simulink model "aerodynamic_hopper"  (R2022b)
settings: Solver=VariableStepAuto  StartTime=0.0  StopTime=1  RelTol=1e-3
libraries: aerolibadyn x1, sharedtransform x1, aerolibasang x1, aerolibatmos2 x1
settings Model: Creator=ks  LastModifiedBy=User
settings OptimizationCC: ReuseModelBlockBuffer=on
settings RTWCC: GPUComputeCapability=5.0

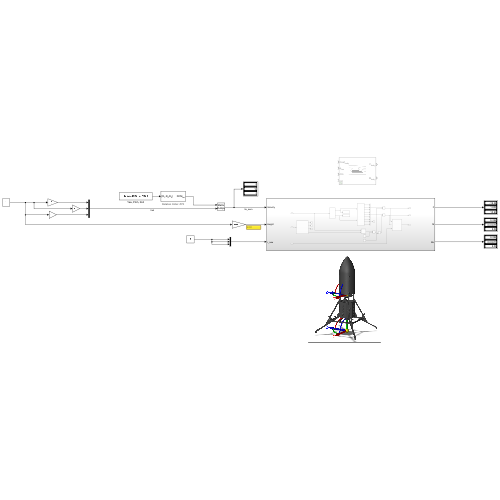
[thumbnail: Simulink's stored preview of the top-level diagram]
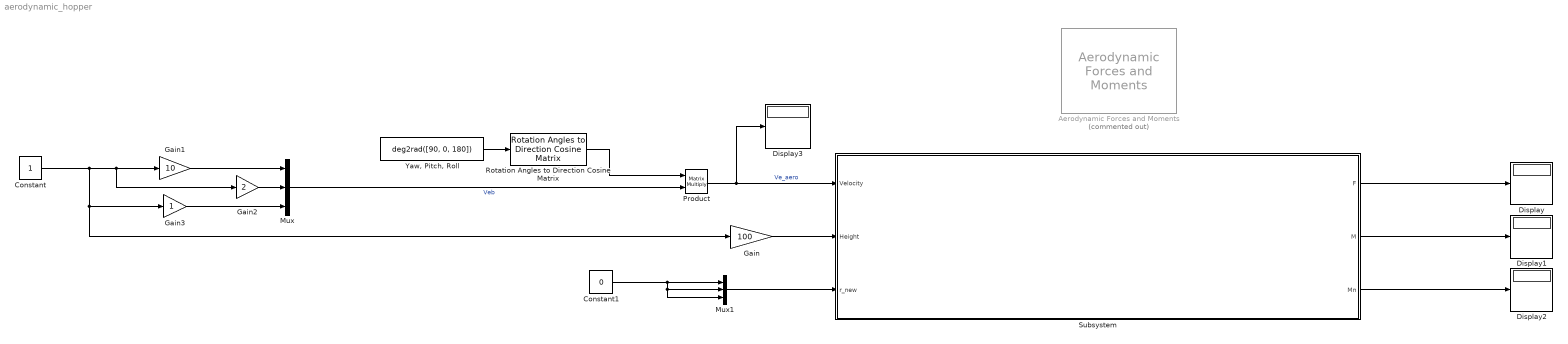
== system aerodynamic_hopper ==
  "Aerodynamic Forces and Moments " : aerolibadyn/Aerodynamic Forces and Moments   Commented=on  inputAxes=Body  outputForceAxes=Body  outputMomentAxes=Body  S=1  b=1  cbar=1
  Constant : Constant
  Constant1 : Constant  Value=0
  Display{,1..3} (4 alike) : Display
  Gain : Gain  Gain=100
  Gain1 : Gain  Gain=10
  Gain2 : Gain  Gain=2
  Gain3 : Gain
  Mux : Mux  Inputs=3
  Mux1 : Mux  Inputs=3
  Product : Product  Multiplication=Matrix(*)
  Rotation Angles to Direction Cosine Matrix : sharedtransform/Rotation Angles to Direction Cosine Matrix  rotationOrder=ZYX  aMode=aMode
  Subsystem : Subsystem
  "Yaw, Pitch, Roll" : Constant  Value=deg2rad([90, 0, 180])
  wires:
  Constant/1 -> Gain1/1, Gain2/1, Gain3/1, Gain/1
  Mux1/1 -> Subsystem/3(r_new)
  Subsystem/1(F) -> Display/1
  Subsystem/2(M) -> Display1/1
  Subsystem/3(Mn) -> Display2/1
  Mux/1 -> Product/2  "Veb"
  Gain/1 -> Subsystem/2(Height)
  Gain1/1 -> Mux/1
  Gain2/1 -> Mux/2
  Constant1/1 -> Mux1/3, Mux1/2, Mux1/1
  "Yaw, Pitch, Roll"/1 -> Rotation Angles to Direction Cosine Matrix/1
  Product/1 -> Display3/1, Subsystem/1(Velocity)  "Ve_aero"
  Rotation Angles to Direction Cosine Matrix/1 -> Product/1
  Gain3/1 -> Mux/3

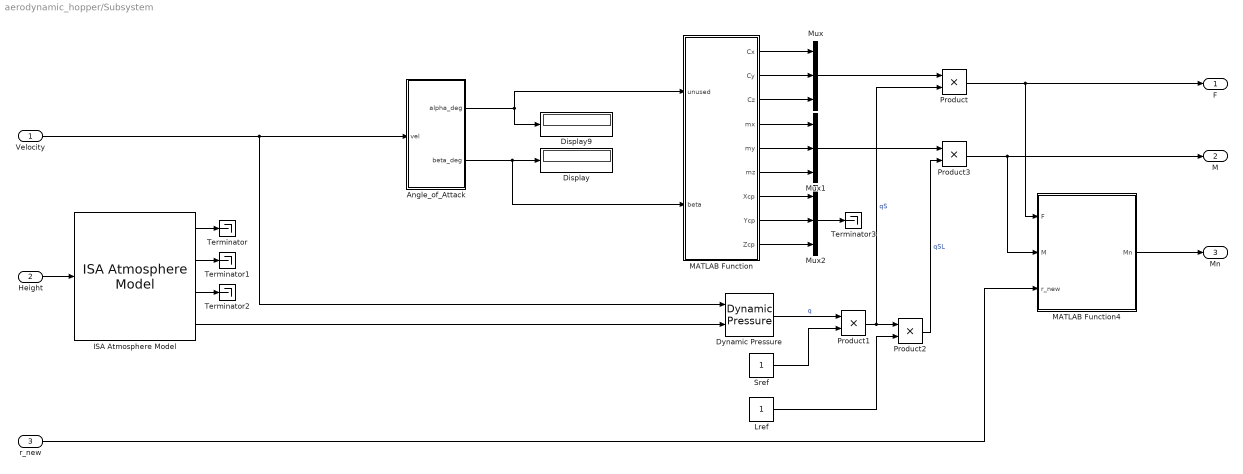
== system aerodynamic_hopper/Subsystem ==
  Velocity : Inport
  Height : Inport  Port=2
  r_new : Inport  Port=3
  Angle_of_Attack : MATLAB Function  TreatAsAtomicUnit=on
  Display : Display
  Display9 : Display
  Dynamic Pressure : aerolibasang/Dynamic Pressure
  ISA Atmosphere Model : aerolibatmos2/ISA Atmosphere Model  custom=off  g=9.80665  gamma=1.4  R=287.0531  L=0.0065  h_trop=11000  h_strat=20000  rho0=1.225  P0=101325  T0=288.15  h0=0
  Lref : Constant
  MATLAB Function : MATLAB Function  TreatAsAtomicUnit=on
  MATLAB Function4 : MATLAB Function  TreatAsAtomicUnit=on
  Mux : Mux  Inputs=3
  Mux1 : Mux  Inputs=3
  Mux2 : Mux  Inputs=3
  Product{,1..3} (4 alike) : Product
  Sref : Constant
  Terminator{,1..3} (4 alike) : Terminator
  F : Outport
  M : Outport  Port=2
  Mn : Outport  Port=3
  wires:
  Mux2/1 -> Terminator3/1
  ISA Atmosphere Model/4 -> Dynamic Pressure/2
  Angle_of_Attack/1(alpha_deg) -> Display9/1, MATLAB Function/1(unused)
  Product/1 -> F/1, MATLAB Function4/1(F)
  MATLAB Function/7(Xcp) -> Mux2/1
  Velocity/1 -> Dynamic Pressure/1, Angle_of_Attack/1(vel)
  Sref/1 -> Product1/2
  r_new/1 -> MATLAB Function4/3(r_new)
  Angle_of_Attack/2(beta_deg) -> Display/1, MATLAB Function/2(beta)
  Product3/1 -> M/1, MATLAB Function4/2(M)
  Mux1/1 -> Product3/1
  MATLAB Function/5(my) -> Mux1/2
  MATLAB Function/3(Cz) -> Mux/3
  ISA Atmosphere Model/3 -> Terminator2/1
  MATLAB Function/6(mz) -> Mux1/3
  Product2/1 -> Product3/2  "qSL"
  Lref/1 -> Product2/2
  ISA Atmosphere Model/2 -> Terminator1/1
  Product1/1 -> Product/2, Product2/1  "qS"
  ISA Atmosphere Model/1 -> Terminator/1
  MATLAB Function/2(Cy) -> Mux/2
  MATLAB Function/1(Cx) -> Mux/1
  MATLAB Function/8(Ycp) -> Mux2/2
  MATLAB Function/9(Zcp) -> Mux2/3
  Dynamic Pressure/1 -> Product1/1  "q"
  Mux/1 -> Product/1
  MATLAB Function/4(mx) -> Mux1/1
  Height/1 -> ISA Atmosphere Model/1
  MATLAB Function4/1(Mn) -> Mn/1

== matlab function aerodynamic_hopper/Subsystem/MATLAB Function ==
  data: unused input; Cx output; beta input; Cy output; Cz output; mx output; my output; mz output; Xcp output; Ycp output; Zcp output
function [Cx, Cy, Cz, mx, my, mz, Xcp, Ycp, Zcp] = fcn(~, beta)

% polynome
Cx =  (6.621e-10)*beta^4 - (4.767e-07)*beta^3 + (9.005e-05)*beta^2 - (0.001687)*beta - 0.2635;
Cy =  9.305e-12*beta^4 - 6.699e-09*beta^3 + 1.502e-06*beta^2 - 0.0001068*beta + 0.01778;
Cz = -5.672e-11*beta^4 - 9.167e-08*beta^3 + 6.192e-05*beta^2 - 0.007794*beta - 0.01447;
mx = -5.921e-11*beta^4 - 2.736e-08*beta^3 + 2.774e-05*beta^2 - 0.003621*beta - 0.03071;
my = -4.569e-13*beta^4 + 6.389e-10*beta^3 - 2.457e-07*beta^2 + 3.404e-05*beta - 0.001447;
mz = -3.350e-10*beta^4 + 2.412e-07*beta^3 - 4.552e-05*beta^2 + 0.0007564*beta + 0.135;

Xcp = -2.414e-27*beta^5 - 5.594e-11*beta^4 + 4.028e-08*beta^3 - 7.294e-06*beta^2 + 1.577e-05*beta + 0.02797;
Ycp = 4.361e-26*beta^5 - 7.658e-11*beta^4 + 5.514e-08*beta^3 - 1.281e-05*beta^2 + 0.00104*beta + 0.5224;
Zcp = -2.884e-13*beta^5 + 2.622e-10*beta^4 - 7.37e-08*beta^3 + 5.553e-06*beta^2 + 8.565e-05*beta + 0.01452;


% X point to the tip of the hopper
% Y 
% Cx =  9.305e-12*beta^4 - 6.699e-09*beta^3 + 1.502e-06*beta^2 - 0.0001068*beta + 0.01778;
% Cy =  6.621e-10*beta^4 - 4.767e-07*beta^3 + 9.005e-05*beta^2 - 0.001687*beta - 0.2635;
% Cz =  5.672e-11*beta^4 + 9.167e-08*beta^3 - 6.192e-05*beta^2 + 0.007794*beta + 0.01447;
% mx = -4.569e-13*beta^4 + 6.389e-10*beta^3 - 2.457e-07*beta^2 + 3.404e-05*beta - 0.001447;
% my = -5.921e-11*beta^4 - 2.736e-08*beta^3 + 2.774e-05*beta^2 - 0.003621*beta - 0.03071;
% mz =  3.350e-10*beta^4 - 2.412e-07*beta^3 + 4.552e-05*beta^2 - 0.0007564*beta - 0.135;
% 
% Xcp = 4.361e-26*beta^5 - 7.658e-11*beta^4 + 5.514e-08*beta^3 - 1.281e-05*beta^2 + 0.00104*beta + 0.5224;
% Ycp = -2.414e-27*beta^5 - 5.594e-11*beta^4 + 4.028e-08*beta^3 - 7.294e-06*beta^2 + 1.577e-05*beta + 0.02797;
% Zcp = 1.665e-13*beta^5 - 1.649e-10*beta^4 + 4.669e-08*beta^3 - 2.495e-06*beta^2 - 0.0002078*beta - 0.01372;

== matlab function aerodynamic_hopper/Subsystem/Angle_of_Attack ==
  data: vel input; alpha_deg output; beta_deg output
function [alpha_deg, beta_deg] = vel2AoA(vel)
% FCN вычисляет угол атаки (alpha) и угол скольжения (beta)
% входы:
%   Vx, Vy, Vz — проекции вектора скорости в системе осей ЛА (м/с)
% выходы:
%   alpha_deg — угол атаки в градусах
%   beta_deg  — угол скольжения в градусах

v = norm(vel);

% Защита от деления на ноль
if v < 1e-10
    alpha_deg = 0.0;
    beta_deg = 0.0;
    return
end

   
alpha_deg = rad2deg(atan2(vel(2), vel(1)));

if vel(2) == 0
    alpha_deg = 0;
end

beta_deg = rad2deg(atan2(vel(3), vel(1)));

if beta_deg < 0
    beta_deg = beta_deg + 360;
end

== matlab function aerodynamic_hopper/Subsystem/MATLAB Function4 ==
  data: F input; M input; Mn output; r_new input
function Mn = fcn(F, M, r_new)

Mn = M - cross(r_new, F);
